simulink subsystem "PieroControladoVPIz"  (R2023b)
settings: Solver=VariableStepAuto  StartTime=0.0  StopTime=10.0  RelTol=1e-3
settings Model: Creator=Hajar  LastModifiedBy=Hajar

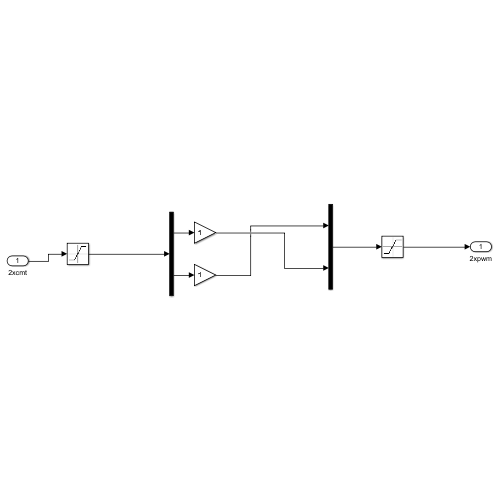
[thumbnail: Simulink's stored preview of the top-level diagram]
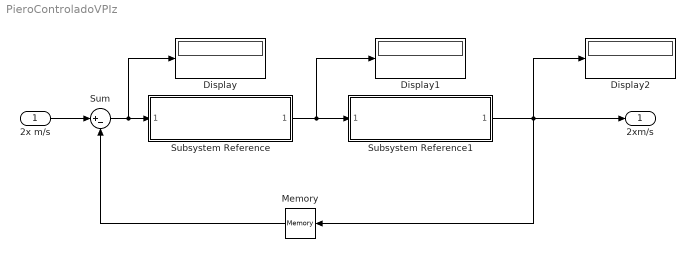
== system PieroControladoVPIz ==
  2x m/s : Inport
  Display : Display
  Display1 : Display
  Display2 : Display
  Memory : Memory
  Subsystem Reference : Subsystem  ReferencedSubsystem=ConroladorPIz
  Subsystem Reference1 : Subsystem  ReferencedSubsystem=PieroHFz
  Sum : Sum  Inputs=|+-
  2xm/s : Outport
  wires:
  Subsystem Reference/1 -> Display1/1, Subsystem Reference1/1
  Subsystem Reference1/1 -> 2xm/s/1, Memory/1, Display2/1
  Memory/1 -> Sum/2
  Sum/1 -> Display/1, Subsystem Reference/1
  2x m/s/1 -> Sum/1
